simulink model "electric_motor_w_inductance"  (R2016b)
settings: Solver=FixedStepAuto  StartTime=0.0  StopTime=10.0  FixedStep=0.001  RelTol=1e-3
values from neighbouring files (symbols this model uses):
  b = 0.00513710988005    [exp1234_estimated_parameters.mat]    (also in exp123_estimated_parameters.mat = 0.00708301164632; exp3_estimated_parameters.mat = 0.015214111895; exp3_estimated_parameters2.mat = 0.0114899753562; motor_calculated_parameters.mat = 0.0173555097)
  beta = 0.000873619169313    [exp1234_estimated_parameters.mat]    (also in exp123_estimated_parameters.mat = 0.000840675695047; exp3_estimated_parameters.mat = 0.000887479829086; exp3_estimated_parameters2.mat = 0.000474777840732; motor_calculated_parameters.mat = 0.000149678)
  J = 0.00106248635811    [exp1234_estimated_parameters.mat]    (also in exp123_estimated_parameters.mat = 0.0010108834441; exp3_estimated_parameters.mat = 0.00123090750882; exp3_estimated_parameters2.mat = 0.000928195104658; motor_calculated_parameters.mat = 0.00123078313678)
  L = 0.0223627298688    [exp1234_estimated_parameters.mat]    (also in exp123_estimated_parameters.mat = 0.0244107453163; exp3_estimated_parameters.mat = 0.000999998484609; exp3_estimated_parameters2.mat = 0.000999998484609; motor_calculated_parameters.mat = 0.001)
  R = 2.45072469052    [exp1234_estimated_parameters.mat]    (also in exp123_estimated_parameters.mat; exp3_estimated_parameters.mat = 1.83400285093; exp3_estimated_parameters2.mat; motor_calculated_parameters.mat = 2.39)
undefined symbols (not defined in the file): i_N, omega_N, u_N
settings Model: Creator=piotr  LastModifiedBy=piotr

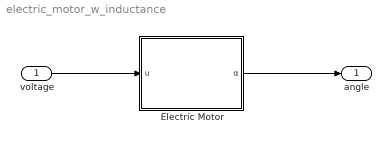
== system electric_motor_w_inductance ==
  voltage : Inport
  Electric Motor : Subsystem  mask{R=R, L=L, K=(u_N-R*i_N)/omega_N, beta=beta, b=b, J=J}
      mask prompts: R "Electrical resistance [Ω]"; L "Motor inductance [H]"; K "Motor constant"; beta "Motor viscous damping [N*m*s/rad]"; b "Motor dry damping [N*m]"; J "Motor moment of inertia [kg*m^2]"
  angle : Outport
  wires:
  voltage/1 -> Electric Motor/1(u)
  Electric Motor/1(α) -> angle/1

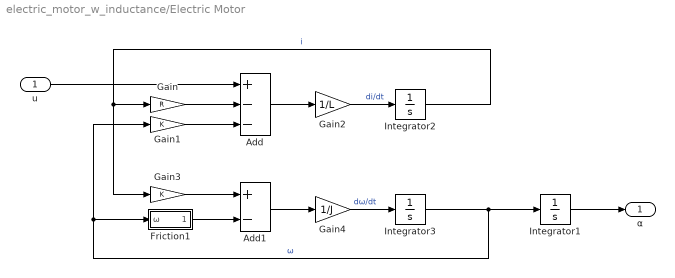
== system electric_motor_w_inductance/Electric Motor ==
  u : Inport
  Add : Sum  Inputs=+--
  Add1 : Sum  Inputs=+-
  Friction1 : Subsystem
  Gain : Gain  Gain=R
  Gain1 : Gain  Gain=K
  Gain2 : Gain  Gain=1/L
  Gain3 : Gain  Gain=K
  Gain4 : Gain  Gain=1/J
  Integrator1 : Integrator
  Integrator2 : Integrator
  Integrator3 : Integrator
  α : Outport
  wires:
  u/1 -> Add/1
  Integrator1/1 -> α/1
  Gain/1 -> Add/2
  Gain1/1 -> Add/3
  Add/1 -> Gain2/1
  Gain2/1 -> Integrator2/1  "di/dt"
  Integrator2/1 -> Gain3/1, Gain/1  "i"
  Friction1/1(Out1) -> Add1/2
  Gain3/1 -> Add1/1
  Add1/1 -> Gain4/1
  Gain4/1 -> Integrator3/1  "dω/dt"
  Integrator3/1 -> Integrator1/1, Friction1/1(ω), Gain1/1  "ω"

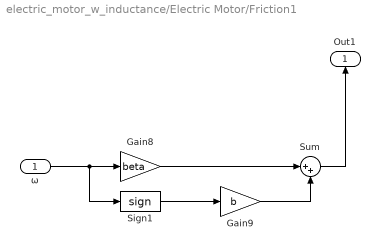
== system electric_motor_w_inductance/Electric Motor/Friction1 ==
  ω : Inport
  Gain8 : Gain  Gain=beta
  Gain9 : Gain  Gain=b
  Sign1 : Signum  ZeroCross=off
  Sum : Sum  Inputs=|++
  Out1 : Outport
  wires:
  Gain9/1 -> Sum/2
  Sum/1 -> Out1/1
  Gain8/1 -> Sum/1
  Sign1/1 -> Gain9/1
  ω/1 -> Gain8/1, Sign1/1
